simulink model "FILTER"  (R2023b)
settings: Solver=VariableStepAuto  StartTime=0.0  StopTime=10.0  RelTol=1e-3
settings Model: Creator=lucaerviati  LastModifiedBy=monis
settings OptimizationCC: ReuseModelBlockBuffer=off

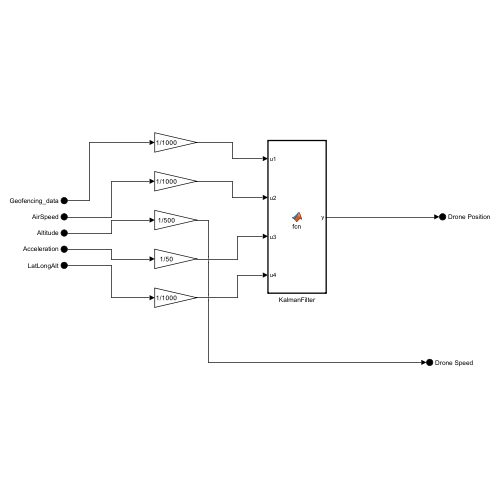
[thumbnail: Simulink's stored preview of the top-level diagram]
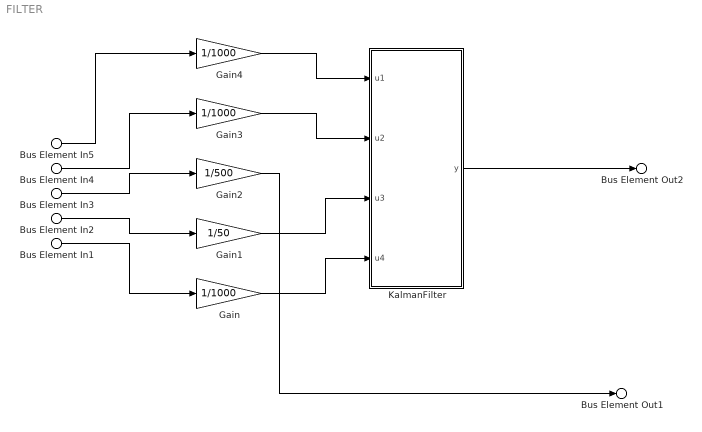
== system FILTER ==
  Bus Element In5 : Inport  PortName=Geofencing_data
  Bus Element In4 : Inport  Port=2  PortName=AirSpeed
  Bus Element In3 : Inport  Port=3  PortName=Altitude
  Bus Element In2 : Inport  Port=4  PortName=Acceleration
  Bus Element In1 : Inport  Port=5  PortName=LatLongAlt
  Gain : Gain  Gain=1/1000
  Gain1 : Gain  Gain=1/50
  Gain2 : Gain  Gain=1/500
  Gain3 : Gain  Gain=1/1000
  Gain4 : Gain  Gain=1/1000
  KalmanFilter : MATLAB Function  TreatAsAtomicUnit=on
  Bus Element Out1 : Outport  PortName=Drone Speed
  Bus Element Out2 : Outport  Port=2  PortName=Drone Position
  wires:
  Bus Element In1/1 -> Gain/1
  Bus Element In2/1 -> Gain1/1
  Bus Element In3/1 -> Gain2/1
  Bus Element In4/1 -> Gain3/1
  Bus Element In5/1 -> Gain4/1
  Gain2/1 -> Bus Element Out1/1
  Gain/1 -> KalmanFilter/4(u4)
  Gain1/1 -> KalmanFilter/3(u3)
  Gain3/1 -> KalmanFilter/2(u2)
  Gain4/1 -> KalmanFilter/1(u1)
  KalmanFilter/1(y) -> Bus Element Out2/1

== matlab function FILTER/KalmanFilter ==
  data: u1 input; y output; u2 input; u3 input; u4 input
function y = fcn(u1, u2, u3, u4)
u = [u1+u2+u3+u4];
y = u;
